simulink model "compare_sat_transfer"  (R2018b)
settings: Solver=VariableStepAuto  StartTime=0.0  StopTime=50  RelTol=1e-3
settings Model: Creator=alexandre  LastModifiedBy=alexandre

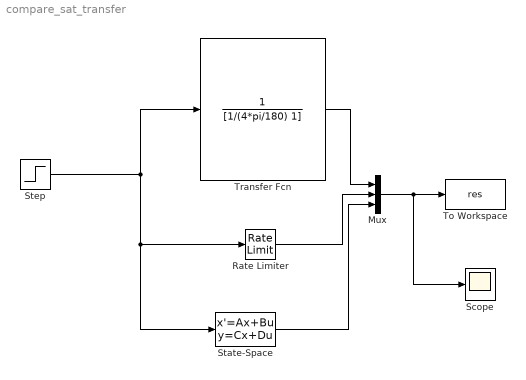
== system compare_sat_transfer ==
  Mux : Mux  Inputs=3
  Rate Limiter : RateLimiter  RisingSlewLimit=4*pi/180  FallingSlewLimit=-4*pi/180  SampleTimeMode=inherited
  Scope : Scope
  State-Space : StateSpace  A=-4*pi/180  B=4*pi/180  D=0  InitialCondition=0
  Step : Step  SampleTime=0.01
  To Workspace : ToWorkspace  VariableName=res  SaveFormat=Timeseries  SampleTime=-1
  Transfer Fcn : TransferFcn  Denominator=[1/(4*pi/180) 1]
  wires:
  Mux/1 -> Scope/1, To Workspace/1
  Rate Limiter/1 -> Mux/2
  Step/1 -> State-Space/1, Rate Limiter/1, Transfer Fcn/1
  State-Space/1 -> Mux/3
  Transfer Fcn/1 -> Mux/1
